simulink model "req19"  (R2019a)
settings: Solver=FixedStepAuto  StartTime=0.0  StopTime=100  RelTol=1e-3
libraries: simulink x10
settings Model: Creator=e40014285  LastModifiedBy=e40014285
settings ConfigComp: CovScope=ReferencedModels  CovHTMLOptions=-sRT=1 -sVT=0 -aTS=1 -bRG=1 -bTC=1 -hTR=0 -nFC=0 -nFD=1 -scm=1 -bcm=1 -xEv=0 -xEM=0  CovHtmlReporting=on  CovCumulativeReport=on  DVMaxProcessTime=6000  DVModelCoverageObjectives=EnhancedMCDC  DVTestSuiteOptimization=Auto  DVDetectOutOfBounds=on  DVReportPDFFormat=on  DVRebuildModelRepresentation=Always

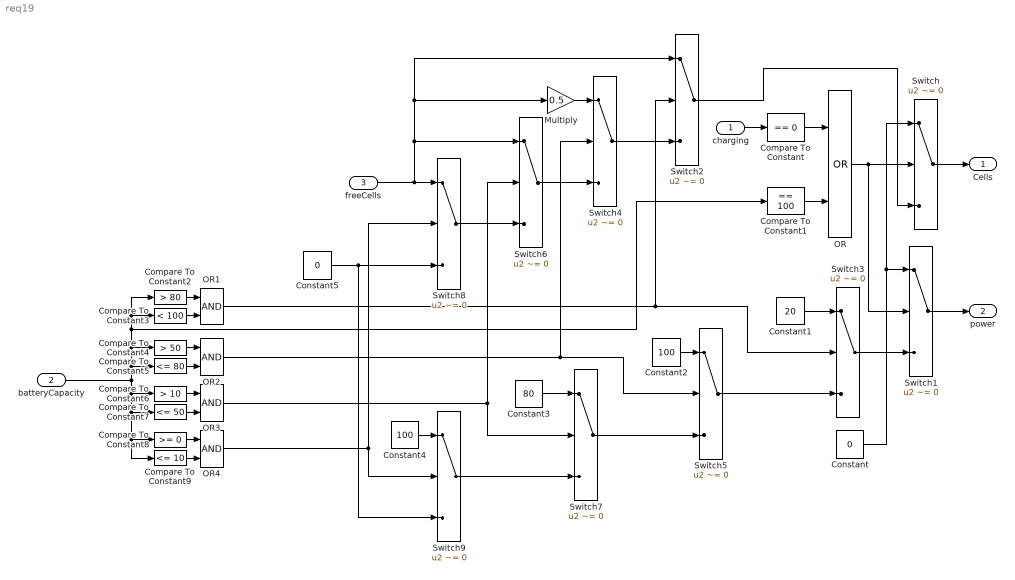
== system req19 ==
  charging : Inport
  batteryCapacity : Inport  Port=2
  freeCells : Inport  Port=3
  Compare To Constant : simulink/Logic and Bit Operations/Compare To Constant  relop===  const=0  OutDataTypeStr=boolean
  Compare To Constant1 : simulink/Logic and Bit Operations/Compare To Constant  relop===  const=100  OutDataTypeStr=boolean
  Compare To Constant2 : simulink/Logic and Bit Operations/Compare To Constant  relop=>  const=80  OutDataTypeStr=boolean
  Compare To Constant3 : simulink/Logic and Bit Operations/Compare To Constant  relop=<  const=100  OutDataTypeStr=boolean
  Compare To Constant4 : simulink/Logic and Bit Operations/Compare To Constant  relop=>  const=50  OutDataTypeStr=boolean
  Compare To Constant5 : simulink/Logic and Bit Operations/Compare To Constant  relop=<=  const=80  OutDataTypeStr=boolean
  Compare To Constant6 : simulink/Logic and Bit Operations/Compare To Constant  relop=>  const=10  OutDataTypeStr=boolean
  Compare To Constant7 : simulink/Logic and Bit Operations/Compare To Constant  relop=<=  const=50  OutDataTypeStr=boolean
  Compare To Constant8 : simulink/Logic and Bit Operations/Compare To Constant  relop=>=  const=0  OutDataTypeStr=boolean
  Compare To Constant9 : simulink/Logic and Bit Operations/Compare To Constant  relop=<=  const=10  OutDataTypeStr=boolean
  Constant : Constant  Value=0
  Constant1 : Constant  Value=20
  Constant2 : Constant  Value=100
  Constant3 : Constant  Value=80
  Constant4 : Constant  Value=100
  Constant5 : Constant  Value=0
  Multiply : Gain  Gain=0.5
  OR : Logic  Operator=OR  AllPortsSameDT=off  OutDataTypeStr=boolean
  OR{1..4} (4 alike) : Logic  AllPortsSameDT=off  OutDataTypeStr=boolean
  Switch{,1..9} (10 alike) : Switch  Criteria=u2 ~= 0
  Cells : Outport
  power : Outport  Port=2
  wires:
  Switch9/1 -> Switch7/3
  OR4/1 -> Switch9/2, Switch8/2
  charging/1 -> Compare To Constant/1
  Compare To Constant1/1 -> OR/2
  Compare To Constant3/1 -> OR1/2
  Switch2/1 -> Switch/3
  batteryCapacity/1 -> Compare To Constant1/1, Compare To Constant2/1, Compare To Constant3/1, Compare To Constant4/1, Compare To Constant5/1, Compare To Constant9/1, Compare To Constant8/1, Compare To Constant7/1, Compare To Constant6/1
  Switch/1 -> Cells/1
  Compare To Constant2/1 -> OR1/1
  Switch3/1 -> Switch1/3
  Compare To Constant/1 -> OR/1
  Constant1/1 -> Switch3/1
  Multiply/1 -> Switch4/1
  Constant2/1 -> Switch5/1
  Switch4/1 -> Switch2/3
  freeCells/1 -> Switch2/1, Multiply/1, Switch6/1, Switch8/1
  Switch1/1 -> power/1
  Compare To Constant4/1 -> OR2/1
  Compare To Constant5/1 -> OR2/2
  Switch5/1 -> Switch3/3
  Constant/1 -> Switch/1, Switch1/1
  Compare To Constant7/1 -> OR3/2
  Compare To Constant6/1 -> OR3/1
  Constant3/1 -> Switch7/1
  Switch6/1 -> Switch4/3
  Constant5/1 -> Switch9/3, Switch8/3
  Switch7/1 -> Switch5/3
  Compare To Constant8/1 -> OR4/1
  Constant4/1 -> Switch9/1
  Switch8/1 -> Switch6/3
  Compare To Constant9/1 -> OR4/2
  OR/1 -> Switch/2, Switch1/2
  OR1/1 -> Switch3/2, Switch2/2
  OR2/1 -> Switch4/2, Switch5/2
  OR3/1 -> Switch6/2, Switch7/2
